simulink model "pen_linear_close_compare"  (R2018a)
settings: Solver=VariableStepAuto  StartTime=0.0  StopTime=10.0  RelTol=1e-3
undefined symbols (not defined in the file): A, B, C, coA, coB, coC, K
settings Model: Creator=ros  LastModifiedBy=ros

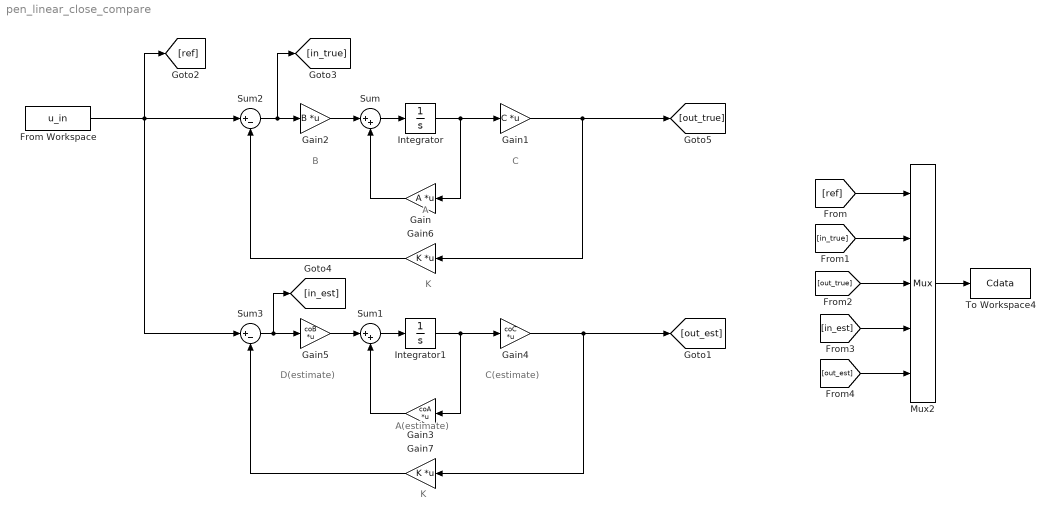
== system pen_linear_close_compare ==
  note: A
  note: A(estimate)
  note: K
  note: K
  note: C(estimate)
  note: D(estimate)
  note: C
  note: B
  From Workspace : FromWorkspace  VariableName=u_in  SampleTime=0.001
  Gain : Gain  Gain=A  Multiplication=Matrix(K*u)
  Gain1 : Gain  Gain=C  Multiplication=Matrix(K*u)
  Gain2 : Gain  Gain=B  Multiplication=Matrix(K*u)
  Gain3 : Gain  Gain=coA  Multiplication=Matrix(K*u)
  Gain4 : Gain  Gain=coC  Multiplication=Matrix(K*u)
  Gain5 : Gain  Gain=coB  Multiplication=Matrix(K*u)
  Gain6 : Gain  Gain=K  Multiplication=Matrix(K*u)
  Gain7 : Gain  Gain=K  Multiplication=Matrix(K*u)
  Integrator : Integrator
  Integrator1 : Integrator
  Mux2 : Mux  Inputs=5
  Sum : Sum  Inputs=|++
  Sum1 : Sum  Inputs=|++
  Sum2 : Sum  Inputs=|+-
  Sum3 : Sum  Inputs=|+-
  To Workspace4 : ToWorkspace  VariableName=Cdata  SaveFormat=Timeseries  SampleTime=-1
  wires:
  Integrator/1 -> Gain1/1, Gain/1
  Gain/1 -> Sum/2
  Gain2/1 -> Sum/1
  Sum/1 -> Integrator/1
  Gain1/1 -> [out_true], Gain6/1
  Mux2/1 -> To Workspace4/1
  Gain3/1 -> Sum1/2
  Sum1/1 -> Integrator1/1
  Integrator1/1 -> Gain4/1, Gain3/1
  Gain5/1 -> Sum1/1
  From Workspace/1 -> [ref], Sum2/1, Sum3/1
  Gain4/1 -> [out_est], Gain7/1
  Gain6/1 -> Sum2/2
  Sum2/1 -> [in_true], Gain2/1
  Gain7/1 -> Sum3/2
  Sum3/1 -> [in_est], Gain5/1
  [ref] -> Mux2/1
  [in_true] -> Mux2/2
  [out_true] -> Mux2/3
  [in_est] -> Mux2/4
  [out_est] -> Mux2/5
